simulink model "vrcrane_joystick"  (Simulink 6.0)
settings: Solver=ode45  StartTime=0.0  StopTime=inf  RelTol=1e-3
PostLoadFcn:
  | Ra=2.6;
  | La=0.012;
  | B=1e-1;
  | Kt=1e2;
  | Kv=3e-2;
  | Kg=1e-3;
  | J=0.1;
  | g=9.80665;
  | m_head=100;
  | Gamma=10;
libraries: vrlib x7, simulink_extras x6
settings Model: Creator=Danek  LastModifiedBy=Danek
settings DataIOCC: SignalLoggingName=logsOut
settings DebuggingCC: CheckExecutionContextPreStartOutputMsg=on  CheckExecutionContextRuntimeOutputMsg=on
settings ModelReferenceCC: UpdateModelReferenceTargets=IfOutOfDate

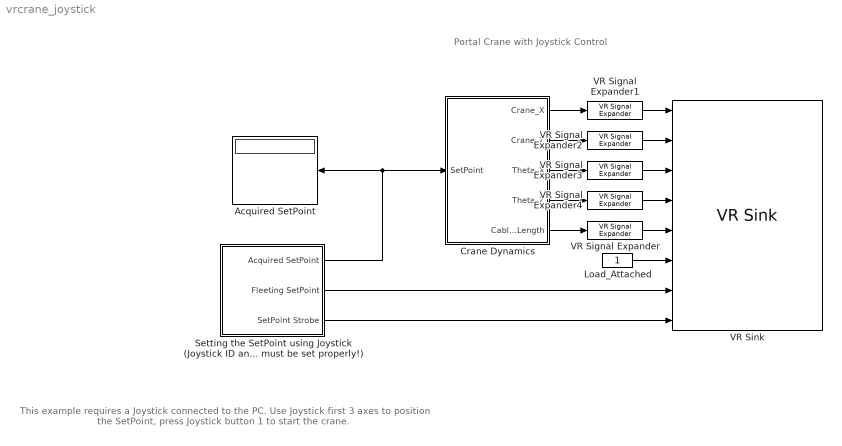
== system vrcrane_joystick ==
  note: Portal Crane with Joystick Control
  note: This example requires a Joystick connected to the PC.
      | Use Joystick first 3 axes to position the SetPoint, press Joystick button 1 to start the crane.
  Acquired SetPoint : Display
  Crane Dynamics : Subsystem  PropExecContextAcrossSSBoundary=on
  Load_Attached : Constant
  "Setting the SetPoint using Joystick (Joystick ID and Axes must be set properly!) " : Subsystem  PropExecContextAcrossSSBoundary=on
  VR Signal Expander : vrlib/VR Signal Expander  outwidth=3  outidx=[2]
  VR Signal Expander1 : vrlib/VR Signal Expander  outwidth=3  outidx=[1]
  VR Signal Expander2 : vrlib/VR Signal Expander  outwidth=3  outidx=[3]
  VR Signal Expander3 : vrlib/VR Signal Expander  outwidth=4  outidx=[4]
  VR Signal Expander4 : vrlib/VR Signal Expander  outwidth=4  outidx=[4]
  VR Sink : vrlib/VR Sink  SampleTime=0.1  ViewEnable=on  RemoteChange=off  RemoteView=off  FieldsWritten=Crane_X.translation.3.1.double#Crane_Z.translation.3.1.double#Parts_Rot_ZAxis.rotation.4.1.double#Parts_Rot_XAxis.rotation.4.1.double#CableUnit.scale.3.1.double#Load_Switch.whichChoice.1.1.double#SetPoint.translation.3.1.double#SP_Highlight.whichChoice.1.1.double  WorldFileName=portal_crane.wrl  WorldDescription=VR Portal Crane  AutoView=on  FigureProperties="{'Position', 'Name', 'Viewpoint', 'CameraBound', 'CameraDirection', 'CameraPosition', 'CameraUpVector', 'ZoomFactor', 'Antialiasing', 'Headlight', 'Lighting', 'NavPanel', 'StatusBar', 'ToolBar', 'Textures', 'Transparency', 'Wireframe', 'NavZones', 'NavMode', 'NavSpeed', 'Record2DCompressMethod', 'Record2DCompressQuality', 'Record2D', 'Record2DFileName'; [6.0000000000000000e+000  7.0000000000000000e+001  5.7600000000000000e+002  3.8000000000000000e+002], 'VR Portal Crane', 'Overview', 'on', [0.0000000000000000e+000  0.0000000000000000e+000 -1.0000000000000000e+000], [0.0000000000000000e+000  0.0000000000000000e+000  0.0000000000000000e+000], [0.0000000000000000e+000  1.0000000000000000e+000  0.0000000000000000e+000], [1.0000000000000000e+000], 'off', 'on', 'on', 'halfbar', 'on', 'on', 'on', 'on', 'off', 'off', 'examine', 'normal', 'auto', [7.5000000000000000e+001], 'off', '%f_anim_%n.avi'}"
  wires:
  "Setting the SetPoint using Joystick (Joystick ID and Axes must be set properly!) "/1(Acquired SetPoint) -> Acquired SetPoint/1, Crane Dynamics/1(SetPoint)
  "Setting the SetPoint using Joystick (Joystick ID and Axes must be set properly!) "/2(Fleeting SetPoint) -> VR Sink/7
  "Setting the SetPoint using Joystick (Joystick ID and Axes must be set properly!) "/3(SetPoint Strobe) -> VR Sink/8
  Load_Attached/1 -> VR Sink/6
  VR Signal Expander/1 -> VR Sink/5
  VR Signal Expander1/1 -> VR Sink/1
  VR Signal Expander2/1 -> VR Sink/2
  VR Signal Expander3/1 -> VR Sink/3
  VR Signal Expander4/1 -> VR Sink/4
  Crane Dynamics/5(Cable_Length) -> VR Signal Expander/1
  Crane Dynamics/1(Crane_X) -> VR Signal Expander1/1
  Crane Dynamics/3(Theta_X) -> VR Signal Expander3/1
  Crane Dynamics/2(Crane_Z) -> VR Signal Expander2/1
  Crane Dynamics/4(Theta_Z) -> VR Signal Expander4/1

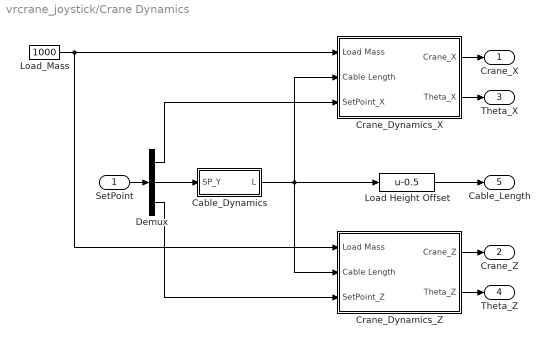
== system vrcrane_joystick/Crane Dynamics ==
  SetPoint : Inport  LatchInput=off
  Cable_Dynamics : Subsystem  PropExecContextAcrossSSBoundary=on
  Crane_Dynamics_X : Subsystem  PropExecContextAcrossSSBoundary=on
  Crane_Dynamics_Z : Subsystem  PropExecContextAcrossSSBoundary=on
  Demux : Demux  Outputs=3
  "Load Height Offset " : Fcn  Expr=u-0.5
  Load_Mass : Constant  Value=1000
  Crane_X : Outport
  Crane_Z : Outport  Port=2
  Theta_X : Outport  Port=3
  Theta_Z : Outport  Port=4
  Cable_Length : Outport  Port=5
  wires:
  Cable_Dynamics/1(L) -> Crane_Dynamics_X/2(Cable Length), Crane_Dynamics_Z/2(Cable Length), "Load Height Offset "/1
  Demux/2 -> Cable_Dynamics/1(SP_Y)
  Demux/1 -> Crane_Dynamics_X/3(SetPoint_X)
  Load_Mass/1 -> Crane_Dynamics_Z/1(Load Mass), Crane_Dynamics_X/1(Load Mass)
  SetPoint/1 -> Demux/1
  Crane_Dynamics_X/1(Crane_X) -> Crane_X/1
  Crane_Dynamics_X/2(Theta_X) -> Theta_X/1
  "Load Height Offset "/1 -> Cable_Length/1
  Crane_Dynamics_Z/1(Crane_Z) -> Crane_Z/1
  Crane_Dynamics_Z/2(Theta_Z) -> Theta_Z/1
  Demux/3 -> Crane_Dynamics_Z/3(SetPoint_Z)

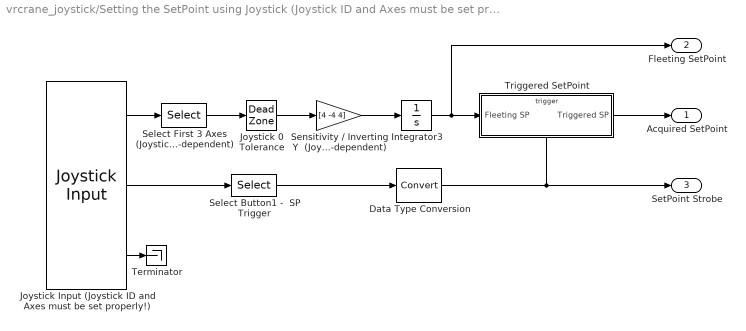
== system vrcrane_joystick/Setting the SetPoint using Joystick (Joystick ID and Axes must be set properly!)  ==
  Data Type Conversion : DataTypeConversion  OutDataTypeMode=boolean
  Integrator3 : Integrator  InitialCondition=[0 0 0]  LimitOutput=on  UpperSaturationLimit=[20 10 20]  LowerSaturationLimit=[0 0 0]
  Joystick 0 Tolerance : DeadZone  LowerValue=-0.2  UpperValue=0.2  SaturateOnIntegerOverflow=on
  Joystick Input (Joystick ID and Axes must be set properly!) : vrlib/Joystick Input  joyid=1  adjustports=off  forcefeed=off
  Select Button1 -  SP Trigger : Selector  Elements=[1]  InputPortWidth=32
  Select First 3 Axes (Joystick -dependent) : Selector  Elements=[1 3 2]  InputPortWidth=8
  Sensitivity / Inverting Y  (Joystick -dependent) : Gain  Gain=[4 -4 4]
  Terminator : Terminator
  Triggered SetPoint : Subsystem  TreatAsAtomicUnit=on  PropExecContextAcrossSSBoundary=on
  Acquired SetPoint : Outport
  Fleeting SetPoint : Outport  Port=2
  SetPoint Strobe : Outport  Port=3
  wires:
  Triggered SetPoint/1(Triggered SP) -> Acquired SetPoint/1
  Joystick Input (Joystick ID and Axes must be set properly!)/1 -> Select First 3 Axes (Joystick -dependent)/1
  Select First 3 Axes (Joystick -dependent)/1 -> Joystick 0 Tolerance/1
  Joystick 0 Tolerance/1 -> Sensitivity / Inverting Y  (Joystick -dependent)/1
  Joystick Input (Joystick ID and Axes must be set properly!)/3 -> Terminator/1
  Joystick Input (Joystick ID and Axes must be set properly!)/2 -> Select Button1 -  SP Trigger/1
  Integrator3/1 -> Fleeting SetPoint/1, Triggered SetPoint/1(Fleeting SP)
  Select Button1 -  SP Trigger/1 -> Data Type Conversion/1
  Sensitivity / Inverting Y  (Joystick -dependent)/1 -> Integrator3/1
  Data Type Conversion/1 -> SetPoint Strobe/1, Triggered SetPoint/Trigger

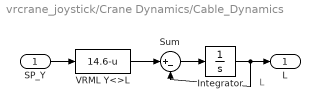
== system vrcrane_joystick/Crane Dynamics/Cable_Dynamics ==
  note: L
  SP_Y : Inport  LatchInput=off
  Integrator : Integrator  InitialCondition=14.6  LimitOutput=on  UpperSaturationLimit=14.6  LowerSaturationLimit=4.6
  Sum : Sum  Inputs=|+-
  VRML Y<>L : Fcn  Expr=14.6-u  SampleTime=0
  L : Outport
  wires:
  Sum/1 -> Integrator/1
  VRML Y<>L/1 -> Sum/1
  Integrator/1 -> Sum/2, L/1
  SP_Y/1 -> VRML Y<>L/1

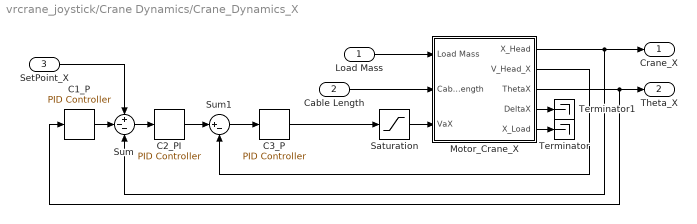
== system vrcrane_joystick/Crane Dynamics/Crane_Dynamics_X ==
  Load Mass : Inport  LatchInput=off
  Cable Length : Inport  Port=2  LatchInput=off
  SetPoint_X : Inport  Port=3  LatchInput=off
  C1_P : simulink_extras/Additional Linear/PID Controller  P=-20  I=0  D=0
  C2_PI : simulink_extras/Additional Linear/PID Controller  P=2.5  I=0  D=0
  C3_P : simulink_extras/Additional Linear/PID Controller  P=5  I=0  D=0
  Motor_Crane_X : Subsystem  PropExecContextAcrossSSBoundary=on
  Saturation : Saturate  UpperLimit=50  LowerLimit=-50
  Sum : Sum  Inputs=+--  SaturateOnIntegerOverflow=on  InputSameDT=on
  Sum1 : Sum  Inputs=|+-  SaturateOnIntegerOverflow=on  InputSameDT=on
  Terminator : Terminator
  Terminator1 : Terminator
  Crane_X : Outport
  Theta_X : Outport  Port=2
  wires:
  Motor_Crane_X/1(X_Head) -> Crane_X/1, Sum/3
  Load Mass/1 -> Motor_Crane_X/1(Load Mass)
  Motor_Crane_X/2(V_Head_X) -> Sum1/2
  Cable Length/1 -> Motor_Crane_X/2(Cable Length)
  Motor_Crane_X/3(ThetaX) -> Theta_X/1, C1_P/1
  Motor_Crane_X/4(DeltaX) -> Terminator1/1
  Motor_Crane_X/5(X_Load) -> Terminator/1
  SetPoint_X/1 -> Sum/1
  Sum/1 -> C2_PI/1
  C2_PI/1 -> Sum1/1
  Sum1/1 -> C3_P/1
  Saturation/1 -> Motor_Crane_X/3(VaX)
  C3_P/1 -> Saturation/1
  C1_P/1 -> Sum/2

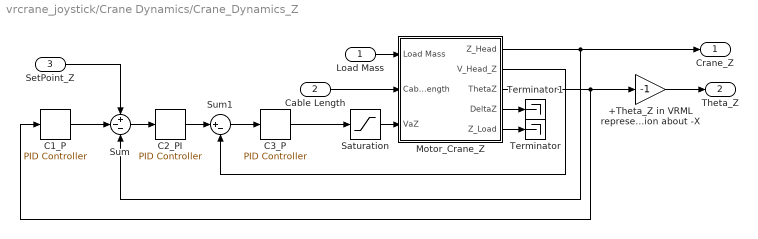
== system vrcrane_joystick/Crane Dynamics/Crane_Dynamics_Z ==
  Load Mass : Inport  LatchInput=off
  Cable Length : Inport  Port=2  LatchInput=off
  SetPoint_Z : Inport  Port=3  LatchInput=off
  +Theta_Z in VRML represented by rotation about -X : Gain  Gain=-1
  C1_P : simulink_extras/Additional Linear/PID Controller  P=-20  I=0  D=0
  C2_PI : simulink_extras/Additional Linear/PID Controller  P=2.5  I=0  D=0
  C3_P : simulink_extras/Additional Linear/PID Controller  P=5  I=0  D=0
  Motor_Crane_Z : Subsystem  PropExecContextAcrossSSBoundary=on
  Saturation : Saturate  UpperLimit=50  LowerLimit=-50
  Sum : Sum  Inputs=+--  SaturateOnIntegerOverflow=on  InputSameDT=on
  Sum1 : Sum  Inputs=|+-  SaturateOnIntegerOverflow=on  InputSameDT=on
  Terminator : Terminator
  Terminator1 : Terminator
  Crane_Z : Outport
  Theta_Z : Outport  Port=2
  wires:
  Motor_Crane_Z/1(Z_Head) -> Crane_Z/1, Sum/3
  Load Mass/1 -> Motor_Crane_Z/1(Load Mass)
  Cable Length/1 -> Motor_Crane_Z/2(Cable Length)
  Motor_Crane_Z/3(ThetaZ) -> +Theta_Z in VRML represented by rotation about -X/1, C1_P/1
  Motor_Crane_Z/4(DeltaZ) -> Terminator1/1
  Motor_Crane_Z/5(Z_Load) -> Terminator/1
  Saturation/1 -> Motor_Crane_Z/3(VaZ)
  C3_P/1 -> Saturation/1
  +Theta_Z in VRML represented by rotation about -X/1 -> Theta_Z/1
  Motor_Crane_Z/2(V_Head_Z) -> Sum1/2
  Sum/1 -> C2_PI/1
  C2_PI/1 -> Sum1/1
  Sum1/1 -> C3_P/1
  C1_P/1 -> Sum/2
  SetPoint_Z/1 -> Sum/1

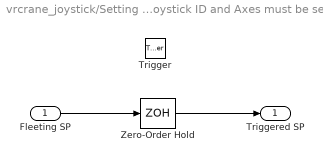
== system vrcrane_joystick/Setting the SetPoint using Joystick (Joystick ID and Axes must be set properly!) /Triggered SetPoint ==
  Fleeting SP : Inport  LatchInput=off
  Trigger : TriggerPort
  Zero-Order Hold : ZeroOrderHold  SampleTime=-1
  Triggered SP : Outport
  wires:
  Zero-Order Hold/1 -> Triggered SP/1
  Fleeting SP/1 -> Zero-Order Hold/1

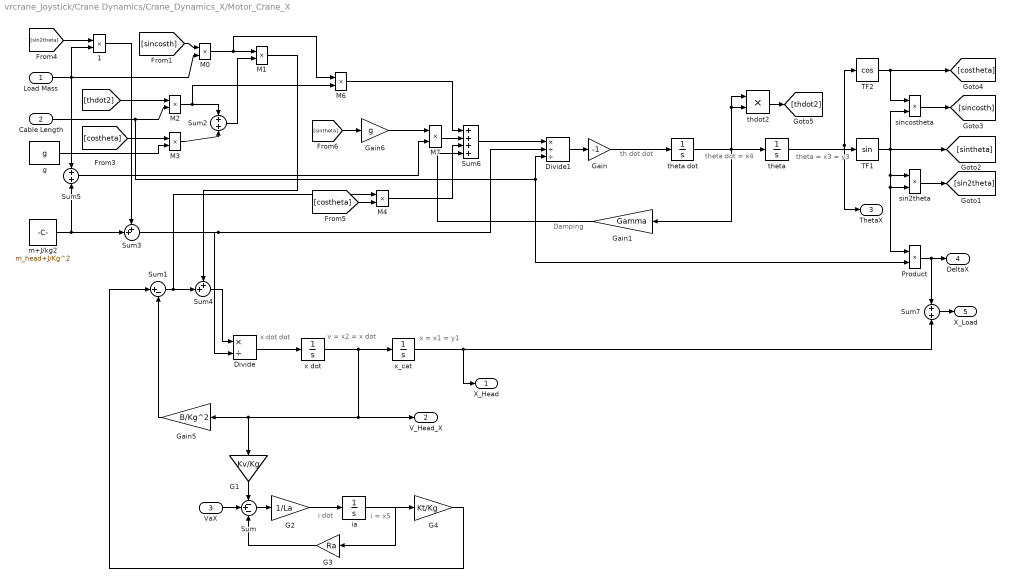
== system vrcrane_joystick/Crane Dynamics/Crane_Dynamics_X/Motor_Crane_X ==
  note: i dot
  note: i = x5
  note: x = x1 = y1
  note: v = x2 = x dot
  note: theta = x3 = y3
  note: theta dot = x4
  note: x dot dot
  note: th dot dot
  note: Damping
  Load Mass : Inport  LatchInput=off
  Cable Length : Inport  Port=2  LatchInput=off
  VaX : Inport  Port=3  LatchInput=off
  " 1" : Product  Inputs=**  OutScaling=2^-10
  Divide : Product  Inputs=*/  OutScaling=2^-10
  Divide1 : Product  Inputs=*//  OutScaling=2^-10
  G1 : Gain  Orientation=down  Gain=Kv/Kg
  G2 : Gain  Gain=1/La
  G3 : Gain  Orientation=left  Gain=Ra
  G4 : Gain  Gain=Kt/Kg
  Gain : Gain  Gain=-1
  Gain1 : Gain  Orientation=left  Gain=Gamma
  Gain5 : Gain  Orientation=left  Gain=B/Kg^2
  Gain6 : Gain  Gain=g
  M{0..4,6..7} (7 alike) : Product  Inputs=**  OutScaling=2^-10
  Product : Product  SaturateOnIntegerOverflow=on
  Sum : Sum  Inputs=-+-
  Sum1 : Sum  Inputs=|+-
  Sum2 : Sum
  Sum3 : Sum  Inputs=++|
  Sum4 : Sum  Inputs=++|
  Sum5 : Sum
  Sum6 : Sum  Inputs=++++
  Sum7 : Sum
  TF1 : Trigonometry
  TF2 : Trigonometry  Operator=cos
  g : Constant  Value=g
  ia : Integrator
  m+J/kg2 : Constant  Value=m_head+J/Kg^2
  sin2theta : Product  Inputs=**  OutScaling=2^-10
  sincostheta : Product  Inputs=**  OutScaling=2^-10
  thdot2 : Product  Inputs=**  OutScaling=2^-10
  theta : Integrator
  theta dot : Integrator
  x dot : Integrator
  x_cat : Integrator
  X_Head : Outport
  V_Head_X : Outport  Port=2
  ThetaX : Outport  Port=3
  DeltaX : Outport  Port=4
  X_Load : Outport  Port=5
  wires:
  G1/1 -> Sum/1
  Sum/1 -> G2/1
  G2/1 -> ia/1
  ia/1 -> G3/1, G4/1
  G3/1 -> Sum/3
  x dot/1 -> x_cat/1, G1/1, Gain5/1, V_Head_X/1
  theta/1 -> ThetaX/1, TF1/1, TF2/1
  theta dot/1 -> theta/1, thdot2/2, thdot2/1, Gain1/1
  G4/1 -> Sum1/1
  Divide/1 -> x dot/1
  Gain5/1 -> Sum1/2
  sin2theta/1 -> [sin2theta]
  sincostheta/1 -> [sincosth]
  [sincosth] -> M0/1
  Load Mass/1 -> Sum5/1, M0/2, " 1"/2
  thdot2/1 -> [thdot2]
  M0/1 -> M1/1, M6/1
  [thdot2] -> M2/1
  [costheta] -> M3/1
  g/1 -> M3/2
  M3/1 -> Sum2/2
  Sum2/1 -> M1/2
  [sin2theta] -> " 1"/1
  " 1"/1 -> Sum3/1
  Sum3/1 -> Divide1/2, Divide/2
  Sum4/1 -> Divide/1
  M1/1 -> Sum4/1
  Sum1/1 -> Sum4/2, M4/1
  M2/1 -> Sum2/1, M6/2
  M6/1 -> Sum6/1
  [costheta] -> M4/2
  Sum5/1 -> M7/2
  [sintheta] -> Gain6/1
  Gain6/1 -> M7/1
  M7/1 -> Sum6/2
  M4/1 -> Sum6/3
  Sum6/1 -> Divide1/1
  Cable Length/1 -> M2/2, Divide1/3, Product/2
  Divide1/1 -> Gain/1
  Gain/1 -> theta dot/1
  x_cat/1 -> X_Head/1, Sum7/2
  VaX/1 -> Sum/2
  m+J/kg2/1 -> Sum3/2, Sum5/2
  Product/1 -> DeltaX/1, Sum7/1
  TF2/1 -> [costheta], sincostheta/1
  TF1/1 -> [sintheta], sincostheta/2, sin2theta/2, Product/1, sin2theta/1
  Sum7/1 -> X_Load/1
  Gain1/1 -> Sum6/4

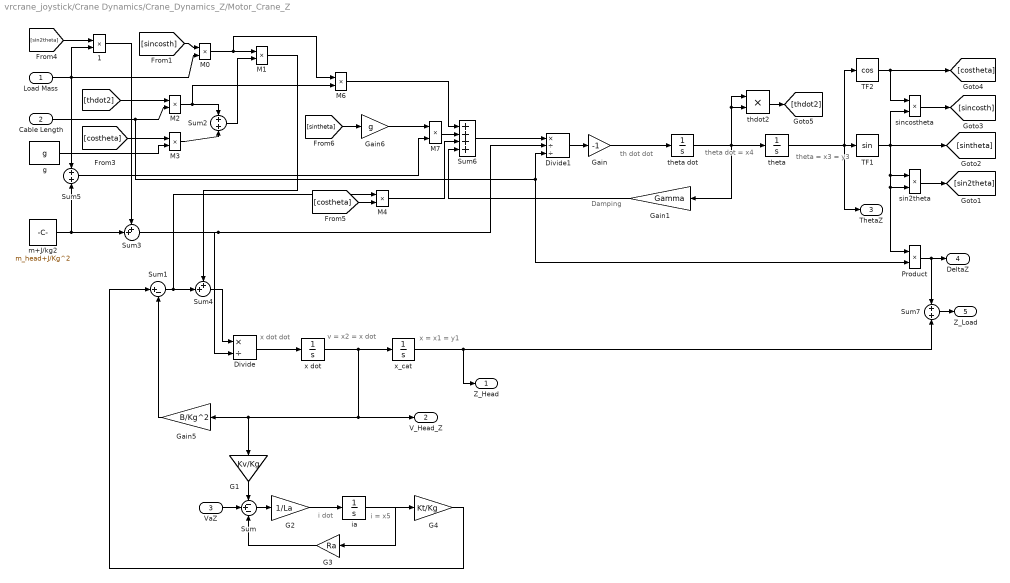
== system vrcrane_joystick/Crane Dynamics/Crane_Dynamics_Z/Motor_Crane_Z ==
  note: i dot
  note: i = x5
  note: x = x1 = y1
  note: v = x2 = x dot
  note: theta = x3 = y3
  note: theta dot = x4
  note: x dot dot
  note: th dot dot
  note: Damping
  Load Mass : Inport  LatchInput=off
  Cable Length : Inport  Port=2  LatchInput=off
  VaZ : Inport  Port=3  LatchInput=off
  " 1" : Product  Inputs=**  OutScaling=2^-10
  Divide : Product  Inputs=*/  OutScaling=2^-10
  Divide1 : Product  Inputs=*//  OutScaling=2^-10
  G1 : Gain  Orientation=down  Gain=Kv/Kg
  G2 : Gain  Gain=1/La
  G3 : Gain  Orientation=left  Gain=Ra
  G4 : Gain  Gain=Kt/Kg
  Gain : Gain  Gain=-1
  Gain1 : Gain  Orientation=left  Gain=Gamma
  Gain5 : Gain  Orientation=left  Gain=B/Kg^2
  Gain6 : Gain  Gain=g
  M{0..4,6..7} (7 alike) : Product  Inputs=**  OutScaling=2^-10
  Product : Product  SaturateOnIntegerOverflow=on
  Sum : Sum  Inputs=-+-
  Sum1 : Sum  Inputs=|+-
  Sum2 : Sum
  Sum3 : Sum  Inputs=++|
  Sum4 : Sum  Inputs=++|
  Sum5 : Sum
  Sum6 : Sum  Inputs=++++
  Sum7 : Sum
  TF1 : Trigonometry
  TF2 : Trigonometry  Operator=cos
  g : Constant  Value=g
  ia : Integrator
  m+J/kg2 : Constant  Value=m_head+J/Kg^2
  sin2theta : Product  Inputs=**  OutScaling=2^-10
  sincostheta : Product  Inputs=**  OutScaling=2^-10
  thdot2 : Product  Inputs=**  OutScaling=2^-10
  theta : Integrator
  theta dot : Integrator
  x dot : Integrator
  x_cat : Integrator
  Z_Head : Outport
  V_Head_Z : Outport  Port=2
  ThetaZ : Outport  Port=3
  DeltaZ : Outport  Port=4
  Z_Load : Outport  Port=5
  wires:
  G1/1 -> Sum/1
  Sum/1 -> G2/1
  G2/1 -> ia/1
  ia/1 -> G3/1, G4/1
  G3/1 -> Sum/3
  x dot/1 -> x_cat/1, G1/1, Gain5/1, V_Head_Z/1
  theta/1 -> ThetaZ/1, TF1/1, TF2/1
  theta dot/1 -> theta/1, thdot2/2, thdot2/1, Gain1/1
  G4/1 -> Sum1/1
  Divide/1 -> x dot/1
  Gain5/1 -> Sum1/2
  sin2theta/1 -> [sin2theta]
  sincostheta/1 -> [sincosth]
  [sincosth] -> M0/1
  Load Mass/1 -> Sum5/1, M0/2, " 1"/2
  thdot2/1 -> [thdot2]
  M0/1 -> M1/1, M6/1
  [thdot2] -> M2/1
  [costheta] -> M3/1
  g/1 -> M3/2
  M3/1 -> Sum2/2
  Sum2/1 -> M1/2
  [sin2theta] -> " 1"/1
  " 1"/1 -> Sum3/1
  Sum3/1 -> Divide1/2, Divide/2
  Sum4/1 -> Divide/1
  M1/1 -> Sum4/1
  Sum1/1 -> Sum4/2, M4/1
  M2/1 -> Sum2/1, M6/2
  M6/1 -> Sum6/1
  [costheta] -> M4/2
  Sum5/1 -> M7/2
  [sintheta] -> Gain6/1
  Gain6/1 -> M7/1
  M7/1 -> Sum6/2
  M4/1 -> Sum6/3
  Sum6/1 -> Divide1/1
  Cable Length/1 -> M2/2, Divide1/3, Product/2
  Divide1/1 -> Gain/1
  Gain/1 -> theta dot/1
  x_cat/1 -> Z_Head/1, Sum7/2
  VaZ/1 -> Sum/2
  m+J/kg2/1 -> Sum3/2, Sum5/2
  Product/1 -> DeltaZ/1, Sum7/1
  TF2/1 -> [costheta], sincostheta/1
  TF1/1 -> [sintheta], sincostheta/2, sin2theta/2, Product/1, sin2theta/1
  Sum7/1 -> Z_Load/1
  Gain1/1 -> Sum6/4
